simulink model "lab_3"  (R2016a)
settings: Solver=VariableStepAuto  StartTime=0.0  StopTime=10.0  RelTol=1e-3
libraries: simulink x2
settings Model: Creator=Anthunder  LastModifiedBy=Anthunder

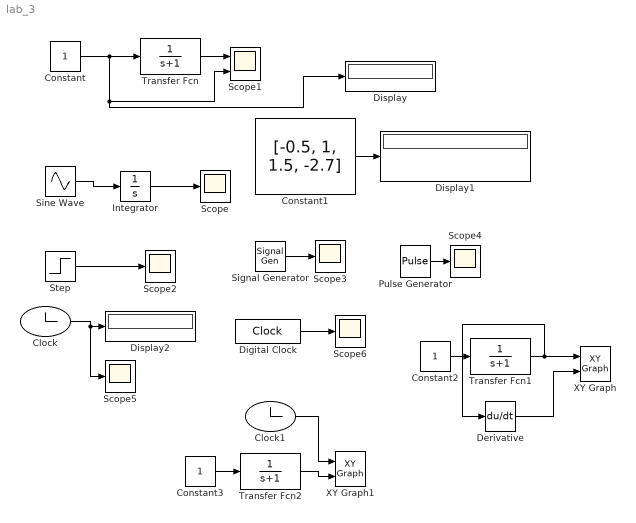
== system lab_3 ==
  Clock : Clock
      settings: Decimation=20
  Clock1 : Clock
      settings: Decimation=20
  Constant : Constant
  Constant1 : Constant  Value=[-0.5, 1, 1.5, -2.7]  VectorParams1D=off
  Constant2 : Constant
  Constant3 : Constant
  Derivative : Derivative
  Digital Clock : DigitalClock
  Display : Display
  Display1 : Display
  Display2 : Display
  Integrator : Integrator
  Pulse Generator : DiscretePulseGenerator  PulseType=Time based  Period=10  PulseWidth=5
  Scope{,2..6} (6 alike) : Scope
  Scope1 : Scope  NumInputPorts=2
  Signal Generator : SignalGenerator  Units=rad/sec
  Sine Wave : Sin  SampleTime=0
  Step : Step  After=10  SampleTime=0
  Transfer Fcn : TransferFcn  Denominator=[1 1]
  Transfer Fcn1 : TransferFcn  Denominator=[1 1]
  Transfer Fcn2 : TransferFcn  Denominator=[1 1]
  XY Graph : simulink/Sinks/XY Graph  xmin=-1  xmax=1  ymin=-1  ymax=1  st=-1
  XY Graph1 : simulink/Sinks/XY Graph  xmin=-1  xmax=1  ymin=-1  ymax=1  st=-1
  wires:
  Constant/1 -> Display/1, Scope1/2, Transfer Fcn/1
  Transfer Fcn/1 -> Scope1/1
  Sine Wave/1 -> Integrator/1
  Integrator/1 -> Scope/1
  Constant1/1 -> Display1/1
  Step/1 -> Scope2/1
  Signal Generator/1 -> Scope3/1
  Pulse Generator/1 -> Scope4/1
  Clock/1 -> Scope5/1, Display2/1
  Digital Clock/1 -> Scope6/1
  Constant2/1 -> Transfer Fcn1/1
  Transfer Fcn1/1 -> XY Graph/1, Derivative/1
  Derivative/1 -> XY Graph/2
  Constant3/1 -> Transfer Fcn2/1
  Clock1/1 -> XY Graph1/1
  Transfer Fcn2/1 -> XY Graph1/2
